simulink model "43_BusNetworkElectricityTransmissionModel"  (R2023b)
settings: Solver=VariableStepAuto  StartTime=0.0  StopTime=0.8  RelTol=1e-3
model workspace (MAT data in the model file):
  BESS_Fp_KDroop = 0.025
  BESS_KSI = 817
  BESS_PWM_fs = 560
  BESS_P_Ki = 0.5
  BESS_P_Kp = 0.0636
  BESS_Pnom = 3000000
  BESS_Q_Ki = 1
  BESS_Q_Kp = 0.0257
  BESS_Vd_Ki = 850
  BESS_Vd_Kp = 0.216
  BESS_Vnom = 1000
  BESS_Vq_KDroop = 0.025
  BESS_Vq_Ki = 850
  BESS_Vq_Kp = 0.216
  Compensation_Ki = 30
  Compensation_Kp = 3
  DC_Ki = 400
  DC_Kp = 8
  F = 0.01
  Flux_min = 0.5
  Grid_Freq_PWM = 2700
  Grid_Ireg_Ki = 5
  Grid_Ireg_Kp = 0.83
  Grid_Ireg_lim = 1.1
  Grid_Modindex_Upper = 1.1
  Grid_conv_Imax = 0.8
  H = 0.685
  Idref_max = 0.9
  Iqref_Tc = 0.3
  Ki_Var = 0.05
  Ki_Vreg = 20
  Ksh = 1.1
  L_pu = 0.3
  Llr = 0.16
  Lls = 0.18
  Lm = 2.9
  LowLoad_P = 130
  Nb_wt = 6
  P_mech = 1080000
  PeakShav_P = 200
  Pitch_Ki = 0
  Pitch_Kp = 150
  Pitch_Max = 27
  Pitch_Tc = 0.01
  Pitch_rate = 10
  Q_Filt = 50
  R_pu = 0.003
  Rotor_Freq_PWM = 1620
  Rotor_Ireg_Ki = 8
  Rotor_Ireg_Kp = 0.6
  Rotor_Ireg_lim = 0.1
  Rotor_Modindex_Upper = 2
  Rr = 0.016
  Rs = 0.023
  SOCBESS : Simulink.Parameter (value not decoded)
  T_set = 0.0001
  Tp = 5e-05
  Ts = 5e-06
  Var_C_Filt = 720000
  Var_reg_max = 1.1
  Var_reg_min = 0.9
  WT_Coeff = [0.645 116 0.4 5 21 0.00912 0.08 0.035]
  WT_H = 4.32
  WT_IGBTRon = 5.931
  WT_Param = [91.204 10143]
  Wind_Freq_Filt = 10000
  Wind_Freq_nom = 60
  Wind_P_nom = 1200000
  Wind_Rotor_V_nom = 1950
  Wind_V_nom = 500
  Zeta_Filt = 0.707106781187
  init = [-0.2 0 0 0 0 0 0 0]
  p = 3
  torque0 = 0.83
  v_Ki = 0.1
  v_Kp = 3.6
  v_Max = 1.2
  v_Min = 0.7
  v_T = 5
  vreg_max = 1
  wind_VDC_nom = 1150
  wt0 = 1.2
undefined symbols (not defined in the file): D1, D11, Delta, DiscIntNeverNeededParam, Iabc, Ion, Lithium, P, Q, Vabc
libraries: powerlib_extras x156, spsSeriesRLCBranchLib x66, spsLoadFlowBusLib x43, spsThreePhaseSeriesRLCLoadLib x33, spsThreePhaseTransformerTwoWindingsLib x32, spsThreePhaseVIMeasurementLib x30, simulink_extras x30, spsDistributedParametersLineLib x22, spsGenericPowerSystemStabilizerLib x20, spsSynchronousMachinepuStandardLib x10, spsExcitationSystemLib x10, spsHydraulicTurbineandGovernorLib x10
(part 9 of 19)

== system 43_BusNetworkElectricityTransmissionModel/ 41.4 MW Wind Generation/41.4 MW Wind Farm/Control System/Control System 3 ==
  Vabc : Inport
  Stator_Iabc : Inport  Port=2
  Grid_Iabc : Inport  Port=3
  Rotor_Iabc : Inport  Port=4
  Vdc_V : Inport  Port=5
  Qref1 : Inport  Port=6
  angle_rotor_rad : Inport  Port=7
  wr : Inport  Port=8
  Bus Creator : BusCreator  Inputs=P,Q
  Constant : Constant  Value=0
  Grid-side Control System : Subsystem
  "Measurement and abc-to-dq transformation " : Subsystem
  PWM Generator (2-Level) : spsPWMGenerator2LevelLib/PWM Generator (2-Level)  ModulatorType=Three-phase bridge (6 pulses)  ModulatorMode=Unsynchronized  Fc=Grid_Freq_PWM  Pc=90  nF=27  MinMax="[ -1  1 ]"  SamplingTechnique=Natural  ModulatingSignals=off  m=0.8  Freq=60  Phase=0  Ts=Ts  ShowCarrierOutport=off
  PWM Generator (2-Level)1 : spsPWMGenerator2LevelLib/PWM Generator (2-Level)  ModulatorType=Three-phase bridge (6 pulses)  ModulatorMode=Unsynchronized  Fc=Rotor_Freq_PWM  Pc=90  nF=27  MinMax="[ -1  1 ]"  SamplingTechnique=Natural  ModulatingSignals=off  m=0.8  Freq=60  Phase=0  Ts=Ts  ShowCarrierOutport=off
  Rotor-side Control System : Subsystem
  Speed & Pitch Control System : Subsystem
  Unit Delay{,2..5} (5 alike) : UnitDelay  SampleTime=Ts  HasFrameUpgradeWarning=on
  Grid_conv_pulses : Outport
  Rotor_conv_pulses : Outport  Port=2
  Pitch : Outport  Port=3
  PQ : Outport  Port=4
  wires:
  [Meas_P] -> Speed & Pitch Control System/2(Meas_P)
  "Measurement and abc-to-dq transformation "/1(Stator_Vdq) -> [Stator_Vdq]
  [Meas_Q] -> Unit Delay4/1
  Unit Delay4/1 -> Bus Creator/2  "Q"
  "Measurement and abc-to-dq transformation "/2(Stator_Idq) -> [Stator_Idq]
  "Measurement and abc-to-dq transformation "/9(w) -> [w]
  Grid_Iabc/1 -> "Measurement and abc-to-dq transformation "/3(Grid_Iabc)
  Grid-side Control System/1(Grid_conv_V) -> Unit Delay/1
  Unit Delay5/1 -> PWM Generator (2-Level)1/1
  Unit Delay2/1 -> Pitch/1
  Unit Delay/1 -> PWM Generator (2-Level)/1
  "Measurement and abc-to-dq transformation "/3(Grid_conv_Idq) -> [Grid_Idq]
  Rotor-side Control System/1(Uctrl_rotor_conv) -> Unit Delay5/1
  "Measurement and abc-to-dq transformation "/13(Delta_Rotor_Angle) -> [Delta_rotor_angle]
  PWM Generator (2-Level)/1 -> Grid_conv_pulses/1
  Vabc/1 -> "Measurement and abc-to-dq transformation "/1(Vabc)
  PWM Generator (2-Level)1/1 -> Rotor_conv_pulses/1
  "Measurement and abc-to-dq transformation "/4(Rotor_Idq) -> [Rotor_Idq]
  "Measurement and abc-to-dq transformation "/5(Vdc_meas_V) -> [Meas_VDC]
  angle_rotor_rad/1 -> "Measurement and abc-to-dq transformation "/7(angle_rotor_rad)
  wr/1 -> "Measurement and abc-to-dq transformation "/8(wr)
  "Measurement and abc-to-dq transformation "/7(Meas_Q) -> [Meas_Q]
  Speed & Pitch Control System/2(Pitch (deg)) -> Unit Delay2/1
  Stator_Iabc/1 -> "Measurement and abc-to-dq transformation "/2(Stator_Iabc)
  Speed & Pitch Control System/1(Tem_cmd) -> [Tem_cmd]
  Rotor_Iabc/1 -> "Measurement and abc-to-dq transformation "/4(Rotor_Iabc)
  Vdc_V/1 -> "Measurement and abc-to-dq transformation "/5(Vdc_V)
  Qref1/1 -> "Measurement and abc-to-dq transformation "/6(Qref)
  [wr] -> Speed & Pitch Control System/1(wr1)
  [Meas_P] -> Unit Delay3/1
  Unit Delay3/1 -> Bus Creator/1  "P"
  "Measurement and abc-to-dq transformation "/11("Qref ") -> [Q_ref]
  "Measurement and abc-to-dq transformation "/6(Meas_P) -> [Meas_P]
  "Measurement and abc-to-dq transformation "/12(Theta_PLL) -> [PLL_theta]
  Bus Creator/1 -> PQ/1
  "Measurement and abc-to-dq transformation "/8(Meas_V) -> [Meas_V]
  "Measurement and abc-to-dq transformation "/10("wr ") -> [wr]
  [Stator_Vdq] -> Grid-side Control System/1(Stator_Vdq)
  Constant/1 -> Grid-side Control System/2(Iq_ref)
  [Meas_VDC] -> Grid-side Control System/3(Vdc)
  [Grid_Idq] -> Grid-side Control System/4(Grid_conv_Idq)
  [PLL_theta] -> Grid-side Control System/5(Theta_PLL)
  [w] -> Grid-side Control System/6(w)
  [Rotor_Idq] -> Rotor-side Control System/1(Rotor_Idq)
  [wr] -> Rotor-side Control System/2(wr)
  [Meas_VDC] -> Rotor-side Control System/3(Vdc)
  [Delta_rotor_angle] -> Rotor-side Control System/4(Angle)
  [Q_ref] -> Rotor-side Control System/5(Qref)
  [Meas_Q] -> Rotor-side Control System/6(Meas_Q)
  [Meas_V] -> Rotor-side Control System/7(Meas_V)
  [Stator_Vdq] -> Rotor-side Control System/8(Stator_Vdq)
  [w] -> Rotor-side Control System/9(w)
  [Stator_Idq] -> Rotor-side Control System/10(Stator_Idq)
  [Tem_cmd] -> Rotor-side Control System/11(Tem_cmd)

== system 43_BusNetworkElectricityTransmissionModel/ 41.4 MW Wind Generation/41.4 MW Wind Farm/Control System/Control System 4 ==
  Vabc : Inport
  Stator_Iabc : Inport  Port=2
  Grid_Iabc : Inport  Port=3
  Rotor_Iabc : Inport  Port=4
  Vdc_V : Inport  Port=5
  Qref1 : Inport  Port=6
  angle_rotor_rad : Inport  Port=7
  wr : Inport  Port=8
  Bus Creator : BusCreator  Inputs=P,Q
  Constant : Constant  Value=0
  Grid-side Control System : Subsystem
  "Measurement and abc-to-dq transformation " : Subsystem
  PWM Generator (2-Level) : spsPWMGenerator2LevelLib/PWM Generator (2-Level)  ModulatorType=Three-phase bridge (6 pulses)  ModulatorMode=Unsynchronized  Fc=Grid_Freq_PWM  Pc=90  nF=27  MinMax="[ -1  1 ]"  SamplingTechnique=Natural  ModulatingSignals=off  m=0.8  Freq=60  Phase=0  Ts=Ts  ShowCarrierOutport=off
  PWM Generator (2-Level)1 : spsPWMGenerator2LevelLib/PWM Generator (2-Level)  ModulatorType=Three-phase bridge (6 pulses)  ModulatorMode=Unsynchronized  Fc=Rotor_Freq_PWM  Pc=90  nF=27  MinMax="[ -1  1 ]"  SamplingTechnique=Natural  ModulatingSignals=off  m=0.8  Freq=60  Phase=0  Ts=Ts  ShowCarrierOutport=off
  Rotor-side Control System : Subsystem
  Speed & Pitch Control System : Subsystem
  Unit Delay{,2..5} (5 alike) : UnitDelay  SampleTime=Ts  HasFrameUpgradeWarning=on
  Grid_conv_pulses : Outport
  Rotor_conv_pulses : Outport  Port=2
  Pitch : Outport  Port=3
  PQ : Outport  Port=4
  wires:
  [Meas_P] -> Speed & Pitch Control System/2(Meas_P)
  "Measurement and abc-to-dq transformation "/1(Stator_Vdq) -> [Stator_Vdq]
  [Meas_Q] -> Unit Delay4/1
  Unit Delay4/1 -> Bus Creator/2  "Q"
  "Measurement and abc-to-dq transformation "/2(Stator_Idq) -> [Stator_Idq]
  "Measurement and abc-to-dq transformation "/9(w) -> [w]
  Grid_Iabc/1 -> "Measurement and abc-to-dq transformation "/3(Grid_Iabc)
  Grid-side Control System/1(Grid_conv_V) -> Unit Delay/1
  Unit Delay5/1 -> PWM Generator (2-Level)1/1
  Unit Delay2/1 -> Pitch/1
  Unit Delay/1 -> PWM Generator (2-Level)/1
  "Measurement and abc-to-dq transformation "/3(Grid_conv_Idq) -> [Grid_Idq]
  Rotor-side Control System/1(Uctrl_rotor_conv) -> Unit Delay5/1
  "Measurement and abc-to-dq transformation "/13(Delta_Rotor_Angle) -> [Delta_rotor_angle]
  PWM Generator (2-Level)/1 -> Grid_conv_pulses/1
  Vabc/1 -> "Measurement and abc-to-dq transformation "/1(Vabc)
  PWM Generator (2-Level)1/1 -> Rotor_conv_pulses/1
  "Measurement and abc-to-dq transformation "/4(Rotor_Idq) -> [Rotor_Idq]
  "Measurement and abc-to-dq transformation "/5(Vdc_meas_V) -> [Meas_VDC]
  angle_rotor_rad/1 -> "Measurement and abc-to-dq transformation "/7(angle_rotor_rad)
  wr/1 -> "Measurement and abc-to-dq transformation "/8(wr)
  "Measurement and abc-to-dq transformation "/7(Meas_Q) -> [Meas_Q]
  Speed & Pitch Control System/2(Pitch (deg)) -> Unit Delay2/1
  Stator_Iabc/1 -> "Measurement and abc-to-dq transformation "/2(Stator_Iabc)
  Speed & Pitch Control System/1(Tem_cmd) -> [Tem_cmd]
  Rotor_Iabc/1 -> "Measurement and abc-to-dq transformation "/4(Rotor_Iabc)
  Vdc_V/1 -> "Measurement and abc-to-dq transformation "/5(Vdc_V)
  Qref1/1 -> "Measurement and abc-to-dq transformation "/6(Qref)
  [wr] -> Speed & Pitch Control System/1(wr1)
  [Meas_P] -> Unit Delay3/1
  Unit Delay3/1 -> Bus Creator/1  "P"
  "Measurement and abc-to-dq transformation "/11("Qref ") -> [Q_ref]
  "Measurement and abc-to-dq transformation "/6(Meas_P) -> [Meas_P]
  "Measurement and abc-to-dq transformation "/12(Theta_PLL) -> [PLL_theta]
  Bus Creator/1 -> PQ/1
  "Measurement and abc-to-dq transformation "/8(Meas_V) -> [Meas_V]
  "Measurement and abc-to-dq transformation "/10("wr ") -> [wr]
  [Stator_Vdq] -> Grid-side Control System/1(Stator_Vdq)
  Constant/1 -> Grid-side Control System/2(Iq_ref)
  [Meas_VDC] -> Grid-side Control System/3(Vdc)
  [Grid_Idq] -> Grid-side Control System/4(Grid_conv_Idq)
  [PLL_theta] -> Grid-side Control System/5(Theta_PLL)
  [w] -> Grid-side Control System/6(w)
  [Rotor_Idq] -> Rotor-side Control System/1(Rotor_Idq)
  [wr] -> Rotor-side Control System/2(wr)
  [Meas_VDC] -> Rotor-side Control System/3(Vdc)
  [Delta_rotor_angle] -> Rotor-side Control System/4(Angle)
  [Q_ref] -> Rotor-side Control System/5(Qref)
  [Meas_Q] -> Rotor-side Control System/6(Meas_Q)
  [Meas_V] -> Rotor-side Control System/7(Meas_V)
  [Stator_Vdq] -> Rotor-side Control System/8(Stator_Vdq)
  [w] -> Rotor-side Control System/9(w)
  [Stator_Idq] -> Rotor-side Control System/10(Stator_Idq)
  [Tem_cmd] -> Rotor-side Control System/11(Tem_cmd)

== system 43_BusNetworkElectricityTransmissionModel/400 kV Solar Farm/DC//DC Boost Converter/MPPT/MPPT  ==
  note: This model uses incremental conductance method to get maximum power point
      |
      | when dP/dV=0  where P= V*I
      | -> d(V*I)/dV = I + V*dI/dV = 0
      | -> dI/dV = -I/V
      |
      | The integrator functions to reduce/minimize errors (dI/dV + I/V)
      | Output = duty cycle changes
  PV_Current : Inport
  PV_Voltage : Inport  Port=2
  Switch port : Inport  Port=3
  Constant2 : Constant  Value=0
  Constant3 : Constant  Value=0
  Dead Zone : DeadZone  LowerValue=-0.05  UpperValue=0.05
  Discrete-Time Integrator : DiscreteIntegrator  SampleTime=T_set  LimitOutput=on  UpperSaturationLimit=1  LowerSaturationLimit=-1  ICPrevOutput=DiscIntNeverNeededParam  ICPrevScaledInput=DiscIntNeverNeededParam
  Fourier : spsFourierLib/Fourier  Freq=1/(MPPT_time)  n=1  InInit=[0, 0]  Ts=T_set
  Fourier1 : spsFourierLib/Fourier  Freq=1/(MPPT_time)  n=1  InInit=[0, 0]  Ts=T_set
  Gain : Gain  Gain=5
  Mean : spsMeanLib/Mean  Freq=1/(MPPT_time)  Vinit=0  Ts=T_set
  Mean1 : spsMeanLib/Mean  Freq=1/(MPPT_time)  Vinit=0  Ts=T_set
  Product : Product  Inputs=*/
  Product2 : Product
  Product3 : Product  Inputs=*/
  Saturation : Saturate  UpperLimit=inf  LowerLimit=eps  ZeroCross=off
  Saturation1 : Saturate  UpperLimit=inf  LowerLimit=eps  ZeroCross=off
  Sum : Sum  Inputs=+-
  Sum1 : Sum
  Switch : Switch  Threshold=0.5  SaturateOnIntegerOverflow=off  InputSameDT=off
  Switch1 : Switch  Threshold=0.5  SaturateOnIntegerOverflow=off  InputSameDT=off
  Trigonometric Function : Trigonometry  Operator=cos
  deg-to-rad conversion : Gain  Gain=pi/180
  delta D : Outport
  tag scope: Imean_PV1=global, Vmean_PV1=global
  wires:
  Mean1/1 -> [Vmean_PV1], Saturation1/1
  PV_Voltage/1 -> Mean1/1, Fourier1/1
  Sum/1 -> deg-to-rad conversion/1
  Product/1 -> Product2/1
  Product3/1 -> Sum1/2
  Saturation1/1 -> Product3/2
  Switch port/1 -> Switch/2, Switch1/2
  Mean/1 -> [Imean_PV1], Product3/1
  Dead Zone/1 -> Gain/1
  Fourier/2 -> Sum/1
  Fourier1/1 -> Saturation/1
  Sum1/1 -> Switch/1  "error"
  Constant2/1 -> Switch/3
  Trigonometric Function/1 -> Product2/2
  Gain/1 -> Discrete-Time Integrator/1
  Discrete-Time Integrator/1 -> Switch1/1
  Switch/1 -> Dead Zone/1
  Fourier1/2 -> Sum/2
  Constant3/1 -> Switch1/3
  deg-to-rad conversion/1 -> Trigonometric Function/1
  PV_Current/1 -> Mean/1, Fourier/1
  Product2/1 -> Sum1/1  "dI/dV (PV)"
  Saturation/1 -> Product/2
  Fourier/1 -> Product/1
  Switch1/1 -> delta D/1

== system 43_BusNetworkElectricityTransmissionModel/400 kV Solar Farm/DC//DC Boost Converter1/MPPT/MPPT  ==
  note: This model uses incremental conductance method to get maximum power point
      |
      | when dP/dV=0  where P= V*I
      | -> d(V*I)/dV = I + V*dI/dV = 0
      | -> dI/dV = -I/V
      |
      | The integrator functions to reduce/minimize errors (dI/dV + I/V)
      | Output = duty cycle changes
  PV_Current : Inport
  PV_Voltage : Inport  Port=2
  Switch port : Inport  Port=3
  Constant2 : Constant  Value=0
  Constant3 : Constant  Value=0
  Dead Zone : DeadZone  LowerValue=-0.05  UpperValue=0.05
  Discrete-Time Integrator : DiscreteIntegrator  SampleTime=T_set  LimitOutput=on  UpperSaturationLimit=1  LowerSaturationLimit=-1  ICPrevOutput=DiscIntNeverNeededParam  ICPrevScaledInput=DiscIntNeverNeededParam
  Fourier : spsFourierLib/Fourier  Freq=1/(MPPT_time)  n=1  InInit=[0, 0]  Ts=T_set
  Fourier1 : spsFourierLib/Fourier  Freq=1/(MPPT_time)  n=1  InInit=[0, 0]  Ts=T_set
  Gain : Gain  Gain=5
  Mean : spsMeanLib/Mean  Freq=1/(MPPT_time)  Vinit=0  Ts=T_set
  Mean1 : spsMeanLib/Mean  Freq=1/(MPPT_time)  Vinit=0  Ts=T_set
  Product : Product  Inputs=*/
  Product2 : Product
  Product3 : Product  Inputs=*/
  Saturation : Saturate  UpperLimit=inf  LowerLimit=eps  ZeroCross=off
  Saturation1 : Saturate  UpperLimit=inf  LowerLimit=eps  ZeroCross=off
  Sum : Sum  Inputs=+-
  Sum1 : Sum
  Switch : Switch  Threshold=0.5  SaturateOnIntegerOverflow=off  InputSameDT=off
  Switch1 : Switch  Threshold=0.5  SaturateOnIntegerOverflow=off  InputSameDT=off
  Trigonometric Function : Trigonometry  Operator=cos
  deg-to-rad conversion : Gain  Gain=pi/180
  delta D : Outport
  tag scope: Imean_PV2=global, Vmean_PV2=global
  wires:
  Mean1/1 -> Saturation1/1
  PV_Voltage/1 -> Mean1/1, Fourier1/1
  Sum/1 -> deg-to-rad conversion/1
  Product/1 -> Product2/1
  Product3/1 -> Sum1/2
  Saturation1/1 -> [Vmean_PV2], Product3/2
  Switch port/1 -> Switch/2, Switch1/2
  Mean/1 -> [Imean_PV2], Product3/1
  Dead Zone/1 -> Gain/1
  Fourier/2 -> Sum/1
  Fourier1/1 -> Saturation/1
  Sum1/1 -> Switch/1  "error"
  Constant2/1 -> Switch/3
  Trigonometric Function/1 -> Product2/2
  Gain/1 -> Discrete-Time Integrator/1
  Discrete-Time Integrator/1 -> Switch1/1
  Switch/1 -> Dead Zone/1
  Fourier1/2 -> Sum/2
  Constant3/1 -> Switch1/3
  deg-to-rad conversion/1 -> Trigonometric Function/1
  PV_Current/1 -> Mean/1, Fourier/1
  Product2/1 -> Sum1/1  "dI/dV (PV)"
  Saturation/1 -> Product/2
  Fourier/1 -> Product/1
  Switch1/1 -> delta D/1

== system 43_BusNetworkElectricityTransmissionModel/400 kV Solar Farm/DC//DC Boost Converter2/MPPT/MPPT  ==
  note: This model uses incremental conductance method to get maximum power point
      |
      | when dP/dV=0  where P= V*I
      | -> d(V*I)/dV = I + V*dI/dV = 0
      | -> dI/dV = -I/V
      |
      | The integrator functions to reduce/minimize errors (dI/dV + I/V)
      | Output = duty cycle changes
  PV_Current : Inport
  PV_Voltage : Inport  Port=2
  Switch port : Inport  Port=3
  Constant2 : Constant  Value=0
  Constant3 : Constant  Value=0
  Dead Zone : DeadZone  LowerValue=-0.05  UpperValue=0.05
  Discrete-Time Integrator : DiscreteIntegrator  SampleTime=T_set  LimitOutput=on  UpperSaturationLimit=1  LowerSaturationLimit=-1  ICPrevOutput=DiscIntNeverNeededParam  ICPrevScaledInput=DiscIntNeverNeededParam
  Display : Display
  Fourier : spsFourierLib/Fourier  Freq=1/(MPPT_time)  n=1  InInit=[0, 0]  Ts=T_set
  Fourier1 : spsFourierLib/Fourier  Freq=1/(MPPT_time)  n=1  InInit=[0, 0]  Ts=T_set
  Gain : Gain  Gain=5
  Mean : spsMeanLib/Mean  Freq=1/(MPPT_time)  Vinit=0  Ts=T_set
  Mean1 : spsMeanLib/Mean  Freq=1/(MPPT_time)  Vinit=0  Ts=T_set
  Product : Product  Inputs=*/
  Product2 : Product
  Product3 : Product  Inputs=*/
  Saturation : Saturate  UpperLimit=inf  LowerLimit=eps  ZeroCross=off
  Saturation1 : Saturate  UpperLimit=inf  LowerLimit=eps  ZeroCross=off
  Sum : Sum  Inputs=+-
  Sum1 : Sum
  Switch : Switch  Threshold=0.5  SaturateOnIntegerOverflow=off  InputSameDT=off
  Switch1 : Switch  Threshold=0.5  SaturateOnIntegerOverflow=off  InputSameDT=off
  Trigonometric Function : Trigonometry  Operator=cos
  deg-to-rad conversion : Gain  Gain=pi/180
  delta D : Outport
  tag scope: Imean_PV3=global, Vmean_PV3=global
  wires:
  Mean1/1 -> Saturation1/1
  PV_Voltage/1 -> Mean1/1, Fourier1/1
  Sum/1 -> deg-to-rad conversion/1
  Product/1 -> Product2/1
  Product3/1 -> Sum1/2
  Saturation1/1 -> [Vmean_PV3], Product3/2
  Switch port/1 -> Switch/2, Switch1/2
  Dead Zone/1 -> Gain/1
  Fourier/2 -> Sum/1
  Fourier1/1 -> Saturation/1
  Sum1/1 -> Switch/1  "error"
  Constant2/1 -> Switch/3
  Trigonometric Function/1 -> Product2/2
  Gain/1 -> Discrete-Time Integrator/1
  Discrete-Time Integrator/1 -> Switch1/1
  Switch/1 -> Dead Zone/1
  Fourier1/2 -> Sum/2
  Constant3/1 -> Switch1/3
  deg-to-rad conversion/1 -> Trigonometric Function/1
  PV_Current/1 -> Mean/1, Fourier/1
  Product2/1 -> Sum1/1  "dI/dV (PV)"
  Saturation/1 -> Product/2
  Fourier/1 -> Product/1
  Switch1/1 -> delta D/1
  Mean/1 -> Display/1, [Imean_PV3], Product3/1

== system 43_BusNetworkElectricityTransmissionModel/400 kV Solar Farm/DC//DC Boost Converter3/MPPT/MPPT  ==
  note: This model uses incremental conductance method to get maximum power point
      |
      | when dP/dV=0  where P= V*I
      | -> d(V*I)/dV = I + V*dI/dV = 0
      | -> dI/dV = -I/V
      |
      | The integrator functions to reduce/minimize errors (dI/dV + I/V)
      | Output = duty cycle changes
  PV_Current : Inport
  PV_Voltage : Inport  Port=2
  Switch port : Inport  Port=3
  Constant2 : Constant  Value=0
  Constant3 : Constant  Value=0
  Dead Zone : DeadZone  LowerValue=-0.05  UpperValue=0.05
  Discrete-Time Integrator : DiscreteIntegrator  SampleTime=T_set  LimitOutput=on  UpperSaturationLimit=1  LowerSaturationLimit=-1  ICPrevOutput=DiscIntNeverNeededParam  ICPrevScaledInput=DiscIntNeverNeededParam
  Fourier : spsFourierLib/Fourier  Freq=1/(MPPT_time)  n=1  InInit=[0, 0]  Ts=T_set
  Fourier1 : spsFourierLib/Fourier  Freq=1/(MPPT_time)  n=1  InInit=[0, 0]  Ts=T_set
  Gain : Gain  Gain=5
  Mean : spsMeanLib/Mean  Freq=1/(MPPT_time)  Vinit=0  Ts=T_set
  Mean1 : spsMeanLib/Mean  Freq=1/(MPPT_time)  Vinit=0  Ts=T_set
  Product : Product  Inputs=*/
  Product2 : Product
  Product3 : Product  Inputs=*/
  Saturation : Saturate  UpperLimit=inf  LowerLimit=eps  ZeroCross=off
  Saturation1 : Saturate  UpperLimit=inf  LowerLimit=eps  ZeroCross=off
  Sum : Sum  Inputs=+-
  Sum1 : Sum
  Switch : Switch  Threshold=0.5  SaturateOnIntegerOverflow=off  InputSameDT=off
  Switch1 : Switch  Threshold=0.5  SaturateOnIntegerOverflow=off  InputSameDT=off
  Trigonometric Function : Trigonometry  Operator=cos
  deg-to-rad conversion : Gain  Gain=pi/180
  delta D : Outport
  tag scope: Imean_PV4=global, Vmean_PV4=global
  wires:
  Mean1/1 -> Saturation1/1
  PV_Voltage/1 -> Mean1/1, Fourier1/1
  Sum/1 -> deg-to-rad conversion/1
  Product/1 -> Product2/1
  Product3/1 -> Sum1/2
  Saturation1/1 -> [Vmean_PV4], Product3/2
  Switch port/1 -> Switch/2, Switch1/2
  Dead Zone/1 -> Gain/1
  Fourier/2 -> Sum/1
  Fourier1/1 -> Saturation/1
  Sum1/1 -> Switch/1  "error"
  Constant2/1 -> Switch/3
  Trigonometric Function/1 -> Product2/2
  Gain/1 -> Discrete-Time Integrator/1
  Discrete-Time Integrator/1 -> Switch1/1
  Switch/1 -> Dead Zone/1
  Fourier1/2 -> Sum/2
  Constant3/1 -> Switch1/3
  deg-to-rad conversion/1 -> Trigonometric Function/1
  PV_Current/1 -> Mean/1, Fourier/1
  Product2/1 -> Sum1/1  "dI/dV (PV)"
  Saturation/1 -> Product/2
  Fourier/1 -> Product/1
  Switch1/1 -> delta D/1
  Mean/1 -> [Imean_PV4], Product3/1

== system 43_BusNetworkElectricityTransmissionModel/Li-ion BESS/BESS/BESS and Controller/BESS ==
  PWM wave : Inport
  Gate_Op : Inport  Port=2
  Battery1 : spsBatteryLib/Battery  BatType=Lithium-Ion  ShowTempParam=off  ThermalPreset="3.6V  2050mAh   (LiCoO2)"  ShowAgeParam=off  NomV=1000  NomQ=3900  SOC=30  Batt_Tr=0.001  PresetModel=on  MaxQ=3900  MinV=750  FullV=1163.9871  Dis_rate=1695.6522  R=0.0025641  Normal_OP=3526.9565  expZone="[1080.3859       191.6087]"  current=[6.5 13 32.5]  Units=Time  Tci=20  NomT=20  T2=-30  MaxQ2=4.8  FullV2=7.1  Normal_OP2=5.655  expZone2="[6.58           1]"  Rca=0.6  ti=2000  Dp=0  Neq0=0  Tsim=1e6  Ta1=25  Qeol=5.4*0.9  Reol=0.013333*1.2  Char_age=[2.3478, 3]  Dis_age=[2.3478, 10]  N1=1500  N2=10500  N3=1000  N4=1400  Ta2=45  N5=950
  Battery2 : spsBatteryLib/Battery  BatType=Lithium-Ion  ShowTempParam=off  ThermalPreset=no  ShowAgeParam=off  NomV=1000  NomQ=3900  SOC=30  Batt_Tr=0.001  PresetModel=on  MaxQ=3900  MinV=750  FullV=1163.9871  Dis_rate=1695.6522  R=0.0025641  Normal_OP=3526.9565  expZone="[1080.3859       191.6087]"  current=[6.5 13 32.5]  Units=Time  Tci=20  NomT=20  T2=-30  MaxQ2=4.8  FullV2=7.1  Normal_OP2=5.655  expZone2="[6.58           1]"  Rca=0.6  ti=2000  Dp=0  Neq0=0  Tsim=1e6  Ta1=25  Qeol=5.4*0.9  Reol=0.013333*1.2  Char_age=[2.3478, 3]  Dis_age=[2.3478, 10]  N1=1500  N2=10500  N3=1000  N4=1400  Ta2=45  N5=950
  Bus Creator : BusCreator  Inputs=2  OutDataTypeStr=Bus: SOC
  Bus Selector : BusSelector  OutputSignals=Gate_P,Gate_N
  Bus Selector1 : BusSelector  OutputSignals=SOC (%)
  Bus Selector2 : BusSelector  OutputSignals=SOC (%)
  Bus Selector3 : BusSelector  OutputSignals=Switch voltage,Switch current
  Bus Selector4 : BusSelector  OutputSignals=Switch voltage,Switch current
  Gain1 : Gain  Gain=1/100
  Gain2 : Gain  Gain=1/100
  IGBT/Diode : spsIGBTDiodeLib/IGBT//Diode  Ron=1e-3  Rs=1e5  Cs=inf  Measurements=on
  IGBT/Diode1 : spsIGBTDiodeLib/IGBT//Diode  Ron=1e-3  Rs=1e5  Cs=inf  Measurements=on
  MINMAX : Subsystem
  Scope : Scope
  Scope1 : Scope  NumInputPorts=2
  Scope2 : Scope
  Scope3 : Scope
  Scope4 : Scope  NumInputPorts=2
  Scope5 : Scope  NumInputPorts=2
  Series RLC Branch : spsSeriesRLCBranchLib/Series RLC Branch  LConnTagsString=__new0  RConnTagsString=__new0  BranchType=C  Resistance=1  Inductance=1e-3  SetiL0=off  InitialCurrent=0  Capacitance=1e-4  Setx0=off  InitialVoltage=0  Measurements=None
  Series RLC Branch1 : spsSeriesRLCBranchLib/Series RLC Branch  LConnTagsString=__new0  RConnTagsString=__new0  BranchType=C  Resistance=1  Inductance=1e-3  SetiL0=off  InitialCurrent=0  Capacitance=1e-4  Setx0=off  InitialVoltage=0  Measurements=None
  Three-Phase V-I Measurement : spsThreePhaseVIMeasurementLib/Three-Phase V-I Measurement  VoltageMeasurement=phase-to-ground  SetLabelV=off  LabelV=Vabc  Vpu=off  VpuLL=off  CurrentMeasurement=yes  SetLabelI=off  LabelI=Iabc  Ipu=off  Pbase=100e6  Vbase=500e3  OutputType=Complex  PhasorSimulation=off  PSBequivalent=0
  Universal Bridge : spsUniversalBridgeLib/Universal Bridge  Arms=3  SnubberResistance=1e5  SnubberCapacitance=inf  Device=IGBT / Diodes  Ron=1e-3  Lon=0  ForwardVoltages="[  0  0  ]"  ForwardVoltage=0  GTOparameters=[ 10e-6 , 20e-6 ]  IGBTparameters=[ 1e-6 , 2e-6 ]  Measurements=None  Measurements_2=None  converterType=Rectifier
  Voltage Measurement : spsVoltageMeasurementLib/Voltage Measurement  PhasorSimulation=off  OutputType=Complex  PSBequivalent=0
  A : PMIOPort  Side=Left
  B : PMIOPort  Port=2  Side=Left
  C : PMIOPort  Port=3  Side=Left
  SOC : Outport
  wires:
  Gate_Op/1 -> Bus Selector/1
  Bus Selector/1 -> [Gate_P]  "<Gate_P>"
  Bus Selector/2 -> [Gate_N]  "<Gate_N>"
  Battery1/1 -> Bus Selector1/1
  Bus Selector1/1 -> Scope2/1, [SoC1]  "<SOC (%)>"
  Bus Selector2/1 -> Scope3/1, [SoC2]  "<SOC (%)>"
  Battery2/1 -> Bus Selector2/1
  [SoC1] -> MINMAX/1(" ")  "MINSOC"
  [SoC2] -> MINMAX/2("  ")  "MAXSOC"
  Bus Creator/1 -> SOC/1
  PWM wave/1 -> Universal Bridge/1
  MINMAX/1(MINSOC) -> Gain2/1  "MINSOC"
  Gain2/1 -> Bus Creator/1  "MINSOC"
  MINMAX/2(MAXSOC) -> Gain1/1  "MAXSOC"
  Gain1/1 -> Bus Creator/2  "MAXSOC"
  [Gate_P] -> IGBT/Diode/1
  [Gate_N] -> IGBT/Diode1/1
  Voltage Measurement/1 -> Scope/1
  Three-Phase V-I Measurement/1 -> Scope1/1
  Three-Phase V-I Measurement/2 -> Scope1/2
  IGBT/Diode/1 -> Bus Selector3/1
  Bus Selector3/2 -> Scope4/2  "<Switch current>"
  Bus Selector3/1 -> Scope4/1  "<Switch voltage>"
  Bus Selector4/2 -> Scope5/2  "<Switch current>"
  IGBT/Diode1/1 -> Bus Selector4/1
  Bus Selector4/1 -> Scope5/1  "<Switch voltage>"
  connections:
  Battery1/LConn1 -- IGBT/Diode/LConn1 -- Voltage Measurement/LConn1
  Battery2/LConn1 -- Battery1/LConn2
  Battery2/LConn2 -- IGBT/Diode1/LConn1 -- Voltage Measurement/LConn2
  Three-Phase V-I Measurement/LConn3 -- Universal Bridge/LConn3
  Universal Bridge/LConn2 -- Three-Phase V-I Measurement/LConn2
  Three-Phase V-I Measurement/LConn1 -- Universal Bridge/LConn1
  C/RConn1 -- Three-Phase V-I Measurement/RConn3
  B/RConn1 -- Three-Phase V-I Measurement/RConn2
  A/RConn1 -- Three-Phase V-I Measurement/RConn1
  Universal Bridge/RConn1 -- IGBT/Diode/RConn1
  IGBT/Diode1/RConn1 -- Universal Bridge/RConn2

== system 43_BusNetworkElectricityTransmissionModel/Li-ion BESS/BESS/BESS and Controller/BESS Control ==
  BMS_BESS : Inport
  Grid_Data : Inport  Port=2
  BESS_Data : Inport  Port=3
  Control : Inport  Port=4
  BESS_Data1 : InportShadow  Port=3
  Bus Selector : BusSelector  OutputSignals=QRef,Command_P
  Bus Selector1 : BusSelector  OutputSignals=Vabc,Iabc
  Bus Selector2 : BusSelector  OutputSignals=P
  Bus Selector3 : BusSelector  OutputSignals=P
  Bus Selector4 : BusSelector  OutputSignals=PRef,PeakShav_Command,BESS_Char_Command
  Constant : Constant  Value=60
  Constant1 : Constant  Value=0.98
  Control1 : InportShadow  Port=4
  Frequency and voltage control : Subsystem
  Peak shaving Mechanism : Subsystem
  PWM_Wave : Outport
  BMS : Outport  Port=2
  BESS_Control : Outport  Port=3
  wires:
  Constant/1 -> Frequency and voltage control/1(f0)
  Constant1/1 -> Frequency and voltage control/2(Vref)
  Peak shaving Mechanism/1(BESS_PRef) -> Frequency and voltage control/3(Pref)
  BMS_BESS/1 -> BESS_Control/1
  Frequency and voltage control/1(PWM_wave) -> PWM_Wave/1
  Peak shaving Mechanism/2(BMS) -> BMS/1
  Control/1 -> Bus Selector/1
  BESS_Data/1 -> Bus Selector1/1
  Bus Selector1/1 -> Frequency and voltage control/4(Iabc)  "<Vabc>"
  Grid_Data/1 -> Bus Selector2/1
  Bus Selector2/1 -> Peak shaving Mechanism/1(P_Grid)  "<P>"
  Bus Selector1/2 -> Frequency and voltage control/5(Vabc)  "<Iabc>"
  Bus Selector/1 -> Frequency and voltage control/6(Qref)  "<QRef>"
  Bus Selector/2 -> Frequency and voltage control/7(powercmd), Frequency and voltage control/8(Powercmd)  "<Command_P>"
  BESS_Data1/1 -> Bus Selector3/1
  Bus Selector3/1 -> Peak shaving Mechanism/3(BESSP)  "<P>"
  Control1/1 -> Bus Selector4/1
  Bus Selector4/1 -> Peak shaving Mechanism/2(BESSPref)  "<PRef>"
  Bus Selector4/2 -> Peak shaving Mechanism/4(PeakShav_Command)  "<PeakShav_Command>"
  Bus Selector4/3 -> Peak shaving Mechanism/5(BESS_Char_Command)  "<BESS_Char_Command>"

== system 43_BusNetworkElectricityTransmissionModel/Li-ion BESS/BESS/BESS and Controller/BMS ==
  BESS_Command : Inport
  Control : Inport  Port=2
  SOC : Inport  Port=3  PortDimensions=2
  BESS Cmd : Subsystem
  Battery Mechanism : Stateflow chart  TreatAsAtomicUnit=on
      settings: PortSchema="{\"entries\":[{\"content\":{\"sides\":[{\"content\":{\"connectorIds\":[\"In1\",\"In2\"]},\"type\":\"ConnectorPlacement.EquallySpacedRectSide\",\"uuid\":\"1be88a38-f019-46bb-9bec-1980b4859a1b\"},{\"content\":{\"connectorIds\":[\"Out1\",\"Out3\",\"Out4\",\"Out2\"],\"side\":\"RIGHT\"},\"type\":\"ConnectorPlacement.EquallySpacedRectSide\",\"uuid\":\"0eec9cfa-e652-46c5-9132-e5d57c4e00b1\"},{\"content\":{\"side\":\"TOP\"},\"type\":\"ConnectorPlacement.EquallySpacedRectSide\",\"uuid\":\"908d2707-0f4b-41e0-b9bc-ca9e7587dd96\"}]},\"type\":\"ConnectorPlacement.EquallySpacedConnector\",\"uuid\":\"7d42ffc8-f308-49ed-bce7-007119405df3\"}],\"packageUris\":[\"http://schema.mathworks.com/mf0/Connector/R2020b\"],\"version\":\"1.0\"}"
  Bus Creator : BusCreator  Inputs=2
  Scope : Scope  NumInputPorts=2
  Scope1 : Scope
  Unit Delay : UnitDelay  SampleTime=-1  HasFrameUpgradeWarning=on
  Unit Delay1 : UnitDelay  SampleTime=-1  HasFrameUpgradeWarning=on
  Gate_Op : Outport
  Stat_BESS : Outport  Port=2
  Stat_SOC : Outport  Port=3
  wires:
  Battery Mechanism/1(Gate_P) -> Scope/1, Unit Delay/1  "Gate_P"
  Battery Mechanism/3(Gate_N) -> Scope/2, Unit Delay1/1  "Gate_N"
  Bus Creator/1 -> Gate_Op/1
  BESS_Command/1 -> BESS Cmd/2(BESS_Command)
  Control/1 -> BESS Cmd/1(Control)
  BESS Cmd/1(Command_BESS) -> Battery Mechanism/2(Command_BESS)
  Unit Delay1/1 -> Bus Creator/2  "Gate_N"
  Unit Delay/1 -> Bus Creator/1  "Gate_P"
  Battery Mechanism/4(Stat_BESS) -> Scope1/1, Stat_BESS/1
  Battery Mechanism/2(Stat_SOC) -> Stat_SOC/1
  SOC/1 -> Battery Mechanism/1(SOC)

== system 43_BusNetworkElectricityTransmissionModel/Li-ion BESS/BESS/BESS and Controller/Inverter Measurement ==
  Bus Creator : BusCreator  Inputs=Vabc,Iabc,P,Q
  Low-Pass Filter (Discrete or Continuous) : eeGeneralControl/Low-Pass Filter (Discrete or Continuous)  K=1  T=0.02  B=inf  A=-inf  init_option=Inherited from block input  x0=0  Ts=Ts
  Low-Pass Filter (Discrete or Continuous)1 : eeGeneralControl/Low-Pass Filter (Discrete or Continuous)  K=1  T=0.02  B=inf  A=-inf  init_option=Inherited from block input  x0=0  Ts=Ts
  Power Calculation : Subsystem
  Scope : Scope
  Three-Phase V-I Measurement : spsThreePhaseVIMeasurementLib/Three-Phase V-I Measurement  VoltageMeasurement=phase-to-ground  SetLabelV=off  LabelV=Vabc  Vpu=off  VpuLL=off  CurrentMeasurement=yes  SetLabelI=off  LabelI=Iabc  Ipu=off  Pbase=100e6  Vbase=500e3  OutputType=Complex  PhasorSimulation=off  PSBequivalent=0
  A : PMIOPort  Side=Left
  B : PMIOPort  Port=2  Side=Left
  C : PMIOPort  Port=3  Side=Left
  A1 : PMIOPort  Port=4  Side=Right
  B1 : PMIOPort  Port=5  Side=Right
  C1 : PMIOPort  Port=6  Side=Right
  BESS_Data : Outport  PortDimensions=8
  wires:
  Three-Phase V-I Measurement/1 -> Power Calculation/1(Vabc), Bus Creator/1  "Vabc"
  Three-Phase V-I Measurement/2 -> Power Calculation/2(Iabc), Bus Creator/2  "Iabc"
  Power Calculation/2(Q) -> Low-Pass Filter (Discrete or Continuous)/1  "Q"
  Bus Creator/1 -> BESS_Data/1
  Power Calculation/1(P) -> Low-Pass Filter (Discrete or Continuous)1/1  "P"
  Low-Pass Filter (Discrete or Continuous)/1 -> Bus Creator/4  "Q"
  Low-Pass Filter (Discrete or Continuous)1/1 -> Scope/1, Bus Creator/3  "P"
  connections:
  Three-Phase V-I Measurement/RConn2 -- B1/RConn1
  Three-Phase V-I Measurement/LConn2 -- B/RConn1
  Three-Phase V-I Measurement/LConn3 -- C/RConn1
  C1/RConn1 -- Three-Phase V-I Measurement/RConn3
  A1/RConn1 -- Three-Phase V-I Measurement/RConn1
  A/RConn1 -- Three-Phase V-I Measurement/LConn1

== system 43_BusNetworkElectricityTransmissionModel/Li-ion BESS/BESS/Grid Measurement/Power Calculation ==
  Vabc : Inport
  Iabc : Inport  Port=2
  " Improved Discrete 3-phase PLL" : Subsystem  mask(Discrete 3-phase PLL){Fmin=0.75*60, Par_Init=[0 60], ParK=[5 3.2 1 50], Ts=Ts}
      mask prompts: Fmin "Minimum frequency (Hz):"; Par_Init "Initial inputs:[ Phase(degrees)   Frequency(Hz) ]"; ParK "Regulator gains [ Kp1 Kp2  Ki1  Ki2 ]"; Ts "Sample time:"
      mask help:
      | This Phase Locked Loop (PLL) system can be used  to synchronize on a set of variable frequency, three-phase sinusoidal signals.
      |
      | Input 1: Vector containing the normalized
      |              three-phase signals [Va Vb Vc]
      | Output 1:  Measured frequency (Hz) = w/(2pi)
      | Output 2:  Ramp w.t   varying between  0 and 2*pi,
      | synchronized on zero crossings of the fundamental (positive-sequence) of phase A.
      | Output 3: Vector [sin(wt) cos(wt)]
      mask init:
      | Kp1=ParK(1);
      | Kp2=ParK(2);
      | Ki1=ParK(3);
      | Ki2=ParK(4);
      | Phase_Init=Par_Init(1);
      | Finit=Par_Init(2);
      | power_initmask();
      settings: OpenFcn=power_openblockproxy();
  "Discrete 3-phase PLL-Driven Positive-Sequence " : Subsystem  mask(Discrete 3-phase PLL-Driven Positive-Sequence Active & Reactive Power){Finit=60, Fmin=45, Par_Vinit=[BESS_Vnom/sqrt(3)*sqrt(2) 30], Par_Iinit=[BESS_Pnom/sqrt(3)/Wind_V_nom*sqrt(2) -10], Ts=Ts}
      mask prompts: Finit "Initial frequency (Hz):"; Fmin "Minimum frequency (Hz):"; Par_Vinit "Voltage initial input: [ Mag  Phase(Degrees) ]"; Par_Iinit "Current initial input: [ Mag  Phase(Degrees) ]"; Ts "Sample time:"
      mask help:
      | This discrete block measures the 3-phase active power P and reactive power Q  associated with a periodic set of 3-phase voltages and currents which may contain harmonics. P and Q are calculated by evaluating the fundamental values (positive-sequence) of the input voltages and currents with a running window over one cycle of the specified frequency (port Freq).
      |  Input port "Sin_Cos" (a two-dimension signal) provides the reference frame required for the computation.
      |
      | input 1: must give the frequency of the fundamental (Hz)
      | Input 2: must contain a  [sin(wt)  cos(wt)] two dimension signal , where w is the rotation speed (rad/s) of the reference frame used for the computation..
      | input 3: Vectorized 3-phase  instantaneous voltage (Vabc)
      | input 4: Vectorized 3-phase instantaneous current (Iabc)
      |
      | Output 1: Vector [Mag_V Mag_I] of the fundamental values (Magnitude) of the voltage & current (peak values of the positive-sequence)
      | Output 2: 3-phase PQ measurement vector [P(W) Q (var)] evaluated at the specified frequency. Current flowing into an RL circuit will produce  positive active and reactive powers.
      |
      | For the first cycle of simulation, the outputs are held constant using the values specified by the parameters "Initial input".
      | he value of the parameter "Minimum frequency" is used to determine the buffer size of the "Variable Transport Delay" block found inside this subsystem.
      mask init:
      | power_initmask();
      settings: OpenFcn=power_openblockproxy();
  Vabc1 : InportShadow
  P : Outport
  Q : Outport  Port=2
  wires:
  Iabc/1 -> "Discrete 3-phase PLL-Driven Positive-Sequence "/4(Iabc_A)
  Vabc/1 -> "Discrete 3-phase PLL-Driven Positive-Sequence "/3(Vabc_V)
  [sin_cos] -> "Discrete 3-phase PLL-Driven Positive-Sequence "/2(Sin_Cos)
  "Discrete 3-phase PLL-Driven Positive-Sequence "/1(Mag_V_V) -> [V_volt]
  "Discrete 3-phase PLL-Driven Positive-Sequence "/2(P_W) -> P/1
  [BESS_Freq] -> "Discrete 3-phase PLL-Driven Positive-Sequence "/1(wind_Freq)
  "Discrete 3-phase PLL-Driven Positive-Sequence "/3(Q_Var) -> Q/1
  Vabc1/1 -> " Improved Discrete 3-phase PLL"/1(Vabc_pu)
  " Improved Discrete 3-phase PLL"/3(Sin_Cos) -> [sin_cos]
  " Improved Discrete 3-phase PLL"/1(wind_Freq) -> [BESS_Freq]
  " Improved Discrete 3-phase PLL"/2(theta) -> [theta]

== system 43_BusNetworkElectricityTransmissionModel/Li-ion BESS/Control/Monitoring and measurement /BESS Measurements ==
  BESS_P : Inport
  BESS_Q : Inport  Port=2
  BESS Voltage : Inport  Port=3
  BESS Current : Inport  Port=4
  BESS Measurements : Subsystem
  wires:
  BESS Voltage/1 -> BESS Measurements/1(Vabc)
  BESS Current/1 -> BESS Measurements/2(Iabc)
  BESS_P/1 -> BESS Measurements/3(BESS _P)
  BESS_Q/1 -> BESS Measurements/4(BESS_Q)

== system 43_BusNetworkElectricityTransmissionModel/Li-ion BESS/Control/Monitoring and measurement /Subsystem ==
  mBESS : Inport
  Constant : Constant
  Less Than : RelationalOperator  Operator=>  OutDataTypeStr=boolean  RndMeth=Simplest  InputSameDT=off
  Out1 : Outport
  wires:
  Less Than/1 -> Out1/1
  Constant/1 -> Less Than/2
  mBESS/1 -> Less Than/1

== system 43_BusNetworkElectricityTransmissionModel/Li-ion BESS/Control/Monitoring and measurement /Subsystem1 ==
  mBESS : Inport
  Constant : Constant
  Less Than : RelationalOperator  Operator=>  OutDataTypeStr=boolean  RndMeth=Simplest  InputSameDT=off
  Out1 : Outport
  wires:
  mBESS/1 -> Less Than/1
  Constant/1 -> Less Than/2
  Less Than/1 -> Out1/1

== system 43_BusNetworkElectricityTransmissionModel/North Network/Regulators 7/Turbine and Excitation Regulators/Stabilitator ==
  Pm : Inport
  Pe : Inport  Port=2
  dw : Inport  Port=3
  Add1 : Sum  Inputs=+-
  Generic Power System Stabilizer : spsGenericPowerSystemStabilizerLib/Generic Power System Stabilizer  Tsensor=30e-3  K=20  Twashout=2  Tleadlag1=[50e-3 20e-3]  Tleadlag2=[3 5.4]  VSlimits=[-0.15 0.15]  Vinit=0  Plot_On=off  MagdB_On=on  FreqRange=logspace(-2,2,500)
      settings: LibrarySourceBlock=|
      | sps_lib/Electrical Machines/Synchronous Machine Control/Generic
      | Power System Stabilizer
  Generic Power System Stabilizer1 : spsGenericPowerSystemStabilizerLib/Generic Power System Stabilizer  Tsensor=30e-3  K=20  Twashout=2  Tleadlag1=[50e-3 20e-3]  Tleadlag2=[3 5.4]  VSlimits=[-0.15 0.15]  Vinit=0  Plot_On=off  MagdB_On=on  FreqRange=logspace(-2,2,500)
      settings: LibrarySourceBlock=|
      | sps_lib/Electrical Machines/Synchronous Machine Control/Generic
      | Power System Stabilizer
  Ground : Ground
  Multiport Switch : MultiPortSwitch  DiagnosticForDefault=None  SaturateOnIntegerOverflow=off  InputSameDT=off
  Out1 : Outport
  wires:
  Pm/1 -> Add1/1
  Generic Power System Stabilizer1/1 -> Multiport Switch/4
  Pe/1 -> Add1/2
  Add1/1 -> Generic Power System Stabilizer/1
  Generic Power System Stabilizer/1 -> Multiport Switch/3
  dw/1 -> Generic Power System Stabilizer1/1
  Ground/1 -> Multiport Switch/2
  [PSS_modes] -> Multiport Switch/1
  Multiport Switch/1 -> Out1/1

== system 43_BusNetworkElectricityTransmissionModel/North Network/Regulators 8/Turbine and Excitation Regulators/Stabilitator ==
  Pm : Inport
  Pe : Inport  Port=2
  dw : Inport  Port=3
  Add1 : Sum  Inputs=+-
  Generic Power System Stabilizer : spsGenericPowerSystemStabilizerLib/Generic Power System Stabilizer  Tsensor=30e-3  K=20  Twashout=2  Tleadlag1=[50e-3 20e-3]  Tleadlag2=[3 5.4]  VSlimits=[-0.15 0.15]  Vinit=0  Plot_On=off  MagdB_On=on  FreqRange=logspace(-2,2,500)
      settings: LibrarySourceBlock=|
      | sps_lib/Electrical Machines/Synchronous Machine Control/Generic
      | Power System Stabilizer
  Generic Power System Stabilizer1 : spsGenericPowerSystemStabilizerLib/Generic Power System Stabilizer  Tsensor=30e-3  K=20  Twashout=2  Tleadlag1=[50e-3 20e-3]  Tleadlag2=[3 5.4]  VSlimits=[-0.15 0.15]  Vinit=0  Plot_On=off  MagdB_On=on  FreqRange=logspace(-2,2,500)
      settings: LibrarySourceBlock=|
      | sps_lib/Electrical Machines/Synchronous Machine Control/Generic
      | Power System Stabilizer
  Ground : Ground
  Multiport Switch : MultiPortSwitch  DiagnosticForDefault=None  SaturateOnIntegerOverflow=off  InputSameDT=off
  Out1 : Outport
  wires:
  Pm/1 -> Add1/1
  Generic Power System Stabilizer1/1 -> Multiport Switch/4
  Pe/1 -> Add1/2
  Add1/1 -> Generic Power System Stabilizer/1
  Generic Power System Stabilizer/1 -> Multiport Switch/3
  dw/1 -> Generic Power System Stabilizer1/1
  Ground/1 -> Multiport Switch/2
  [PSS_modes] -> Multiport Switch/1
  Multiport Switch/1 -> Out1/1

== system 43_BusNetworkElectricityTransmissionModel/North Network/Regulators 9/Turbine and Excitation Regulators/Stabilitator ==
  Pm : Inport
  Pe : Inport  Port=2
  dw : Inport  Port=3
  Add1 : Sum  Inputs=+-
  Generic Power System Stabilizer : spsGenericPowerSystemStabilizerLib/Generic Power System Stabilizer  Tsensor=30e-3  K=20  Twashout=2  Tleadlag1=[50e-3 20e-3]  Tleadlag2=[3 5.4]  VSlimits=[-0.15 0.15]  Vinit=0  Plot_On=off  MagdB_On=on  FreqRange=logspace(-2,2,500)
      settings: LibrarySourceBlock=|
      | sps_lib/Electrical Machines/Synchronous Machine Control/Generic
      | Power System Stabilizer
  Generic Power System Stabilizer1 : spsGenericPowerSystemStabilizerLib/Generic Power System Stabilizer  Tsensor=30e-3  K=20  Twashout=2  Tleadlag1=[50e-3 20e-3]  Tleadlag2=[3 5.4]  VSlimits=[-0.15 0.15]  Vinit=0  Plot_On=off  MagdB_On=on  FreqRange=logspace(-2,2,500)
      settings: LibrarySourceBlock=|
      | sps_lib/Electrical Machines/Synchronous Machine Control/Generic
      | Power System Stabilizer
  Ground : Ground
  Multiport Switch : MultiPortSwitch  DiagnosticForDefault=None  SaturateOnIntegerOverflow=off  InputSameDT=off
  Stab : Outport
  wires:
  Pm/1 -> Add1/1
  Generic Power System Stabilizer1/1 -> Multiport Switch/4
  Pe/1 -> Add1/2
  Add1/1 -> Generic Power System Stabilizer/1
  Generic Power System Stabilizer/1 -> Multiport Switch/3
  dw/1 -> Generic Power System Stabilizer1/1
  Ground/1 -> Multiport Switch/2
  [PSS_modes] -> Multiport Switch/1
  Multiport Switch/1 -> Stab/1

== system 43_BusNetworkElectricityTransmissionModel/South Network/Regulators 1/Turbine and Excitation Regulators/Stabilitator ==
  Pm : Inport
  Pe : Inport  Port=2
  dw : Inport  Port=3
  Add1 : Sum  Inputs=+-
  Generic Power System Stabilizer : spsGenericPowerSystemStabilizerLib/Generic Power System Stabilizer  Tsensor=30e-3  K=20  Twashout=2  Tleadlag1=[50e-3 20e-3]  Tleadlag2=[3 5.4]  VSlimits=[-0.15 0.15]  Vinit=0  Plot_On=off  MagdB_On=on  FreqRange=logspace(-2,2,500)
      settings: LibrarySourceBlock=|
      | sps_lib/Electrical Machines/Synchronous Machine Control/Generic
      | Power System Stabilizer
  Generic Power System Stabilizer1 : spsGenericPowerSystemStabilizerLib/Generic Power System Stabilizer  Tsensor=30e-3  K=20  Twashout=2  Tleadlag1=[50e-3 20e-3]  Tleadlag2=[3 5.4]  VSlimits=[-0.15 0.15]  Vinit=0  Plot_On=off  MagdB_On=on  FreqRange=logspace(-2,2,500)
      settings: LibrarySourceBlock=|
      | sps_lib/Electrical Machines/Synchronous Machine Control/Generic
      | Power System Stabilizer
  Ground : Ground
  Multiport Switch : MultiPortSwitch  DiagnosticForDefault=None  SaturateOnIntegerOverflow=off  InputSameDT=off
  Out1 : Outport
  wires:
  Pm/1 -> Add1/1
  Generic Power System Stabilizer1/1 -> Multiport Switch/4
  Pe/1 -> Add1/2
  Add1/1 -> Generic Power System Stabilizer/1
  Generic Power System Stabilizer/1 -> Multiport Switch/3
  dw/1 -> Generic Power System Stabilizer1/1
  Ground/1 -> Multiport Switch/2
  [PSS_modes] -> Multiport Switch/1
  Multiport Switch/1 -> Out1/1

== system 43_BusNetworkElectricityTransmissionModel/South Network/Regulators 2/Turbine and Excitation Regulators/Stabilitator ==
  Pm : Inport
  Pe : Inport  Port=2
  dw : Inport  Port=3
  Add1 : Sum  Inputs=+-
  Generic Power System Stabilizer : spsGenericPowerSystemStabilizerLib/Generic Power System Stabilizer  Tsensor=30e-3  K=20  Twashout=2  Tleadlag1=[50e-3 20e-3]  Tleadlag2=[3 5.4]  VSlimits=[-0.15 0.15]  Vinit=0  Plot_On=off  MagdB_On=on  FreqRange=logspace(-2,2,500)
      settings: LibrarySourceBlock=|
      | sps_lib/Electrical Machines/Synchronous Machine Control/Generic
      | Power System Stabilizer
  Generic Power System Stabilizer1 : spsGenericPowerSystemStabilizerLib/Generic Power System Stabilizer  Tsensor=30e-3  K=20  Twashout=2  Tleadlag1=[50e-3 20e-3]  Tleadlag2=[3 5.4]  VSlimits=[-0.15 0.15]  Vinit=0  Plot_On=off  MagdB_On=on  FreqRange=logspace(-2,2,500)
      settings: LibrarySourceBlock=|
      | sps_lib/Electrical Machines/Synchronous Machine Control/Generic
      | Power System Stabilizer
  Ground : Ground
  Multiport Switch : MultiPortSwitch  DiagnosticForDefault=None  SaturateOnIntegerOverflow=off  InputSameDT=off
  Out1 : Outport
  wires:
  Pm/1 -> Add1/1
  Generic Power System Stabilizer1/1 -> Multiport Switch/4
  Pe/1 -> Add1/2
  Add1/1 -> Generic Power System Stabilizer/1
  Generic Power System Stabilizer/1 -> Multiport Switch/3
  dw/1 -> Generic Power System Stabilizer1/1
  Ground/1 -> Multiport Switch/2
  [PSS_modes] -> Multiport Switch/1
  Multiport Switch/1 -> Out1/1

== system 43_BusNetworkElectricityTransmissionModel/South Network/Regulators 3/Turbine and Excitation Regulators/Stabilitator ==
  Pm : Inport
  Pe : Inport  Port=2
  dw : Inport  Port=3
  Add1 : Sum  Inputs=+-
  Generic Power System Stabilizer : spsGenericPowerSystemStabilizerLib/Generic Power System Stabilizer  Tsensor=30e-3  K=20  Twashout=2  Tleadlag1=[50e-3 20e-3]  Tleadlag2=[3 5.4]  VSlimits=[-0.15 0.15]  Vinit=0  Plot_On=off  MagdB_On=on  FreqRange=logspace(-2,2,500)
      settings: LibrarySourceBlock=|
      | sps_lib/Electrical Machines/Synchronous Machine Control/Generic
      | Power System Stabilizer
  Generic Power System Stabilizer1 : spsGenericPowerSystemStabilizerLib/Generic Power System Stabilizer  Tsensor=30e-3  K=20  Twashout=2  Tleadlag1=[50e-3 20e-3]  Tleadlag2=[3 5.4]  VSlimits=[-0.15 0.15]  Vinit=0  Plot_On=off  MagdB_On=on  FreqRange=logspace(-2,2,500)
      settings: LibrarySourceBlock=|
      | sps_lib/Electrical Machines/Synchronous Machine Control/Generic
      | Power System Stabilizer
  Ground : Ground
  Multiport Switch : MultiPortSwitch  DiagnosticForDefault=None  SaturateOnIntegerOverflow=off  InputSameDT=off
  Out1 : Outport
  wires:
  Pm/1 -> Add1/1
  Generic Power System Stabilizer1/1 -> Multiport Switch/4
  Pe/1 -> Add1/2
  Add1/1 -> Generic Power System Stabilizer/1
  Generic Power System Stabilizer/1 -> Multiport Switch/3
  dw/1 -> Generic Power System Stabilizer1/1
  Ground/1 -> Multiport Switch/2
  [PSS_modes] -> Multiport Switch/1
  Multiport Switch/1 -> Out1/1

== system 43_BusNetworkElectricityTransmissionModel/South Network/Regulators 4/Turbine and Excitation Regulators/Stabilitator ==
  Pm : Inport
  Pe : Inport  Port=2
  dw : Inport  Port=3
  Add1 : Sum  Inputs=+-
  Generic Power System Stabilizer : spsGenericPowerSystemStabilizerLib/Generic Power System Stabilizer  Tsensor=30e-3  K=20  Twashout=2  Tleadlag1=[50e-3 20e-3]  Tleadlag2=[3 5.4]  VSlimits=[-0.15 0.15]  Vinit=0  Plot_On=off  MagdB_On=on  FreqRange=logspace(-2,2,500)
      settings: LibrarySourceBlock=|
      | sps_lib/Electrical Machines/Synchronous Machine Control/Generic
      | Power System Stabilizer
  Generic Power System Stabilizer1 : spsGenericPowerSystemStabilizerLib/Generic Power System Stabilizer  Tsensor=30e-3  K=20  Twashout=2  Tleadlag1=[50e-3 20e-3]  Tleadlag2=[3 5.4]  VSlimits=[-0.15 0.15]  Vinit=0  Plot_On=off  MagdB_On=on  FreqRange=logspace(-2,2,500)
      settings: LibrarySourceBlock=|
      | sps_lib/Electrical Machines/Synchronous Machine Control/Generic
      | Power System Stabilizer
  Ground : Ground
  Multiport Switch : MultiPortSwitch  DiagnosticForDefault=None  SaturateOnIntegerOverflow=off  InputSameDT=off
  Out1 : Outport
  wires:
  Pm/1 -> Add1/1
  Generic Power System Stabilizer1/1 -> Multiport Switch/4
  Pe/1 -> Add1/2
  Add1/1 -> Generic Power System Stabilizer/1
  Generic Power System Stabilizer/1 -> Multiport Switch/3
  dw/1 -> Generic Power System Stabilizer1/1
  Ground/1 -> Multiport Switch/2
  [PSS_modes] -> Multiport Switch/1
  Multiport Switch/1 -> Out1/1

== system 43_BusNetworkElectricityTransmissionModel/South Network/Regulators 5/Turbine and Excitation Regulators/Stabilitator ==
  Pm : Inport
  Pe : Inport  Port=2
  dw : Inport  Port=3
  Add1 : Sum  Inputs=+-
  Generic Power System Stabilizer : spsGenericPowerSystemStabilizerLib/Generic Power System Stabilizer  Tsensor=30e-3  K=20  Twashout=2  Tleadlag1=[50e-3 20e-3]  Tleadlag2=[3 5.4]  VSlimits=[-0.15 0.15]  Vinit=0  Plot_On=off  MagdB_On=on  FreqRange=logspace(-2,2,500)
      settings: LibrarySourceBlock=|
      | sps_lib/Electrical Machines/Synchronous Machine Control/Generic
      | Power System Stabilizer
  Generic Power System Stabilizer1 : spsGenericPowerSystemStabilizerLib/Generic Power System Stabilizer  Tsensor=30e-3  K=20  Twashout=2  Tleadlag1=[50e-3 20e-3]  Tleadlag2=[3 5.4]  VSlimits=[-0.15 0.15]  Vinit=0  Plot_On=off  MagdB_On=on  FreqRange=logspace(-2,2,500)
      settings: LibrarySourceBlock=|
      | sps_lib/Electrical Machines/Synchronous Machine Control/Generic
      | Power System Stabilizer
  Ground : Ground
  Multiport Switch : MultiPortSwitch  DiagnosticForDefault=None  SaturateOnIntegerOverflow=off  InputSameDT=off
  Out1 : Outport
  wires:
  Pm/1 -> Add1/1
  Generic Power System Stabilizer1/1 -> Multiport Switch/4
  Pe/1 -> Add1/2
  Add1/1 -> Generic Power System Stabilizer/1
  Generic Power System Stabilizer/1 -> Multiport Switch/3
  dw/1 -> Generic Power System Stabilizer1/1
  Ground/1 -> Multiport Switch/2
  [PSS_modes] -> Multiport Switch/1
  Multiport Switch/1 -> Out1/1
